simulink model "ANF"  (R2017b)
settings: Solver=VariableStepAuto  StartTime=0.0  StopTime=0.4  MaxStep=1e-4  RelTol=1e-3
libraries: powerlib x5
settings Model: Creator=Kalpit  LastModifiedBy=Kalpit

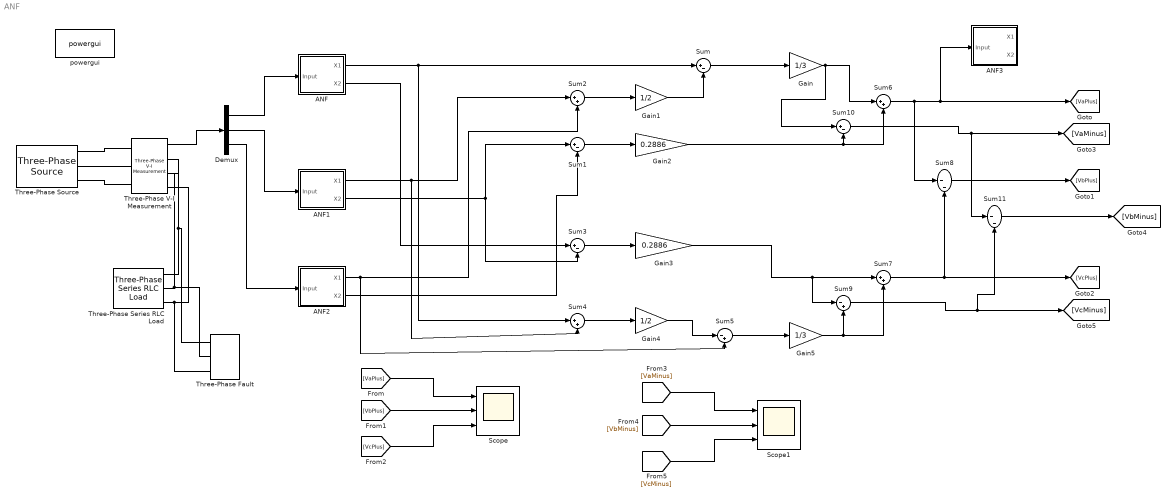
== system ANF ==
  ANF : Subsystem
  ANF1 : Subsystem
  ANF2 : Subsystem
  ANF3 : Subsystem
  Demux : Demux  Outputs=3
  Gain : Gain  Gain=1/3
  Gain1 : Gain  Gain=1/2
  Gain2 : Gain  Gain=0.2886
  Gain3 : Gain  Gain=0.2886
  Gain4 : Gain  Gain=1/2
  Gain5 : Gain  Gain=1/3
  Scope : Scope  NumInputPorts=3
  Scope1 : Scope  NumInputPorts=3
  Sum{,1,3,10} (4 alike) : Sum  Inputs=|+-
  Sum11 : Sum  Inputs=|--
  Sum{2,4,6..7} (4 alike) : Sum  Inputs=|++
  Sum5 : Sum  Inputs=|-+
  Sum8 : Sum  Inputs=|--
  Sum9 : Sum  Inputs=|-+
  Three-Phase Series RLC Load : powerlib/Elements/Three-Phase Series RLC Load  LConnTagsString=A|B|C  Configuration=Y (grounded)  NominalVoltage=415  Vabc=[1e3 1e3 1e3]  Vabcp=[1e3 1e3 1e3]  NominalFrequency=50  UnbalancedPower=off  ActivePower=10e3  InductivePower=100  CapacitivePower=100  Pabc=[10e3 9e3 11e3]  QLabc=[100 90 110]  QCabc=[100 90 110]  Pabcp=[10e3 9e3 11e3]  QLabcp=[100 90 110]  QCabcp=[100 90 110]  Measurements=None  LoadType=constant Z
  Three-Phase V-I Measurement : powerlib/Measurements/Three-Phase V-I Measurement  VoltageMeasurement=phase-to-ground  SetLabelV=off  LabelV=Vabc  Vpu=off  VpuLL=off  CurrentMeasurement=no  SetLabelI=off  LabelI=Iabc  Ipu=off  Pbase=100e6  Vbase=1  OutputType=Complex  PhasorSimulation=off  PSBequivalent=0
  Three-Phase Fault : powerlib/Elements/Three-Phase Fault  InitialStates=0  FaultA=on  FaultB=off  FaultC=on  GroundFault=on  SwitchTimes=0.2  External=off  SwitchStatus=NaN  FaultResistance=0.001  GroundResistance=0.01  SnubberResistance=1e6  SnubberCapacitance=inf  Measurements=None
  Three-Phase Source : powerlib/Electrical Sources/Three-Phase Source  InternalConnection=Yg  VoltagePhases=off  Voltage=415  PhaseAngle=0  Voltage_phases=[25e3 25e3 25e3]/sqrt(3)  PhaseAngles_phases=[0 -120 +120]  Frequency=50  NonIdealSource=on  SpecifyImpedance=off  Resistance=0.8929  Inductance=16.58e-3  ShortCircuitLevel=100e6  BaseVoltage=25e3  XRratio=7  BusType=swing  Pref=10e3  Qref=0  Prefabc=[10e3, 10e3, 10e3]  Qrefabc=[0, 0, 0]  Qmin=-inf  Qmax=inf
  powergui : powerlib/powergui  Priority=1  SimulationMode=Continuous  SampleTime=50e-6  frequency=60  Iterations=50  frequencyindice=50  Pbase=100e6  ErrMax=1e-4  UnitsV=kV  UnitsW=MW  buscounter=0  FunctionMessages=off  echomessages=off  EnableUseOfTLC=off  CurrentSourceSwitches=off  DisableSnubberDevices=off  DisableRonSwitches=off  DisableVfSwitches=off  DisplayEquations=off  SolverType=Tustin/Backward Euler (TBE)  Interpol=off  ExternalGateDelay=off  methode=off  Ts=100  x0status=blocks  SPID=on  SwTol=0  HookPort=off  RestoreLinks=warning  ResistiveCurrentMeasurement=off  Frange=[0:2:500]  Ylog=off  Xlog=on  ShowGrid=off  save=off  variable=ZData  structure=0  ZoomFFT=off  StartTime=0.0  cycles=1  DisplayStyle=1  fundamental=60  FreqAxis=off  MaxFrequency=1000  frequencyindicesteady=1  RmsSteady=1  display=off
  wires:
  Sum/1 -> Gain/1
  Gain1/1 -> Sum/2
  Sum2/1 -> Gain1/1
  ANF1/1(X1) -> Sum4/2, Sum2/1
  ANF/2(X2) -> Sum3/1
  ANF1/2(X2) -> Sum1/1, Sum3/2
  ANF2/1(X1) -> Sum5/2, Sum2/2
  ANF2/2(X2) -> Sum1/2
  Sum1/1 -> Gain2/1
  Sum3/1 -> Gain3/1
  Gain4/1 -> Sum5/1
  Sum5/1 -> Gain5/1
  Sum7/1 -> [VcPlus], Sum8/2
  Gain3/1 -> Sum9/1, Sum7/1
  Gain2/1 -> Sum10/2, Sum6/2
  Gain/1 -> Sum10/1, Sum6/1
  Gain5/1 -> Sum9/2, Sum7/2
  Sum8/1 -> [VbPlus]
  Sum10/1 -> Sum11/1, [VaMinus]
  Sum9/1 -> Sum11/2, [VcMinus]
  Sum11/1 -> [VbMinus]
  Sum4/1 -> Gain4/1
  Demux/1 -> ANF/1(Input)
  Demux/2 -> ANF1/1(Input)
  Demux/3 -> ANF2/1(Input)
  Three-Phase V-I Measurement/1 -> Demux/1
  [VaPlus] -> Scope/1
  [VbPlus] -> Scope/2
  [VcPlus] -> Scope/3
  ANF/1(X1) -> Sum4/1, Sum/1
  [VcMinus] -> Scope1/3
  [VbMinus] -> Scope1/2
  [VaMinus] -> Scope1/1
  Sum6/1 -> Sum8/1, ANF3/1(Input), [VaPlus]
  connections:
  Three-Phase V-I Measurement/LConn2 -- Three-Phase Source/RConn2
  Three-Phase Source/RConn1 -- Three-Phase V-I Measurement/LConn1
  Three-Phase Source/RConn3 -- Three-Phase V-I Measurement/LConn3
  Three-Phase Series RLC Load/LConn1 -- Three-Phase Fault/LConn1 -- Three-Phase V-I Measurement/RConn1
  Three-Phase V-I Measurement/RConn2 -- Three-Phase Fault/LConn2 -- Three-Phase Series RLC Load/LConn2
  Three-Phase V-I Measurement/RConn3 -- Three-Phase Fault/LConn3 -- Three-Phase Series RLC Load/LConn3

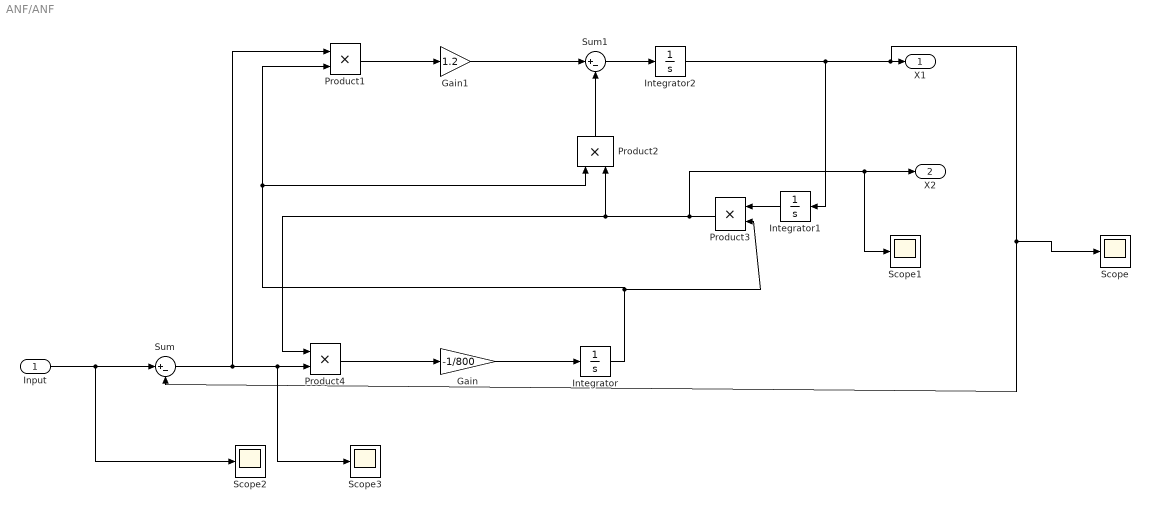
== system ANF/ANF ==
  Input : Inport
  Gain : Gain  Gain=-1/800
  Gain1 : Gain  Gain=1.2
  Integrator : Integrator  InitialCondition=100*pi
  Integrator1 : Integrator
  Integrator2 : Integrator
  Product{1..4} (4 alike) : Product
  Scope{,1..3} (4 alike) : Scope
  Sum : Sum  Inputs=|+-
  Sum1 : Sum  Inputs=|+-
  X1 : Outport
  X2 : Outport  Port=2
  wires:
  Sum1/1 -> Integrator2/1
  Sum/1 -> Product1/1, Scope3/1, Product4/2
  Product4/1 -> Gain/1
  Input/1 -> Scope2/1, Sum/1
  Integrator1/1 -> Product3/1
  Integrator2/1 -> Scope/1, Sum/2, X1/1, Integrator1/1
  Integrator/1 -> Product3/2, Product2/1, Product1/2
  Product3/1 -> Scope1/1, X2/1, Product4/1, Product2/2
  Product1/1 -> Gain1/1
  Product2/1 -> Sum1/2
  Gain/1 -> Integrator/1
  Gain1/1 -> Sum1/1

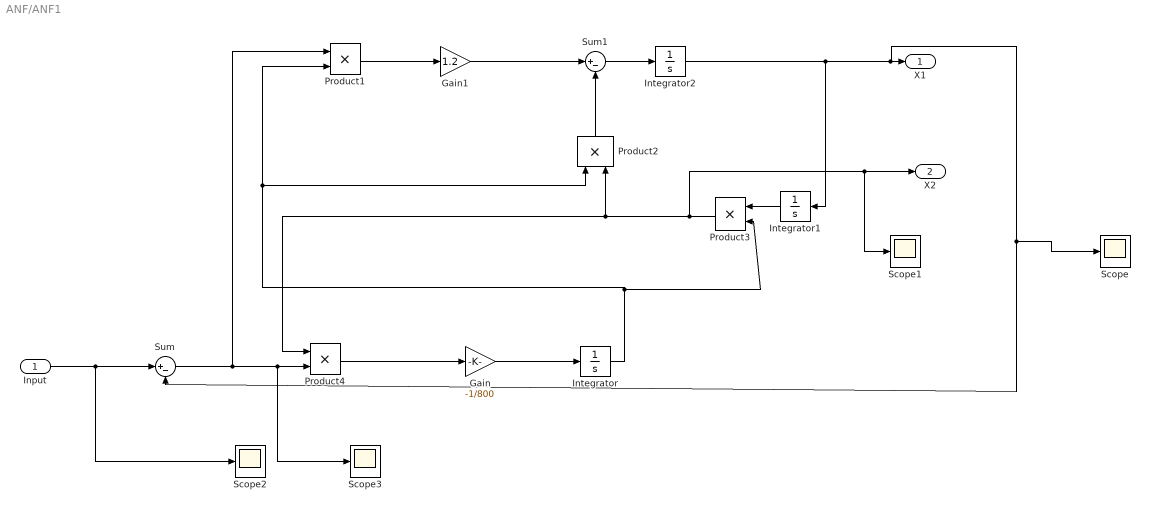
== system ANF/ANF1 ==
  Input : Inport
  Gain : Gain  Gain=-1/800
  Gain1 : Gain  Gain=1.2
  Integrator : Integrator  InitialCondition=100*pi - (2*pi/3)
  Integrator1 : Integrator
  Integrator2 : Integrator
  Product{1..4} (4 alike) : Product
  Scope{,1..3} (4 alike) : Scope
  Sum : Sum  Inputs=|+-
  Sum1 : Sum  Inputs=|+-
  X1 : Outport
  X2 : Outport  Port=2
  wires:
  Gain1/1 -> Sum1/1
  Gain/1 -> Integrator/1
  Product2/1 -> Sum1/2
  Product1/1 -> Gain1/1
  Product3/1 -> Product2/2, Product4/1, X2/1, Scope1/1
  Integrator/1 -> Product1/2, Product2/1, Product3/2
  Integrator2/1 -> Integrator1/1, X1/1, Sum/2, Scope/1
  Integrator1/1 -> Product3/1
  Input/1 -> Sum/1, Scope2/1
  Product4/1 -> Gain/1
  Sum/1 -> Product4/2, Scope3/1, Product1/1
  Sum1/1 -> Integrator2/1

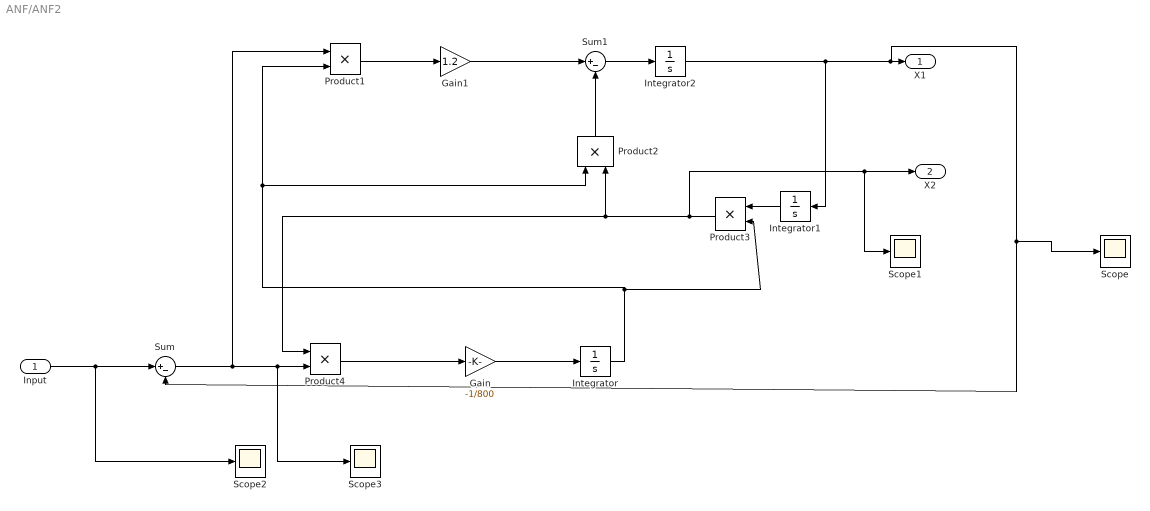
== system ANF/ANF2 ==
  Input : Inport
  Gain : Gain  Gain=-1/800
  Gain1 : Gain  Gain=1.2
  Integrator : Integrator  InitialCondition=100*pi + (2*pi/3)
  Integrator1 : Integrator
  Integrator2 : Integrator
  Product{1..4} (4 alike) : Product
  Scope{,1..3} (4 alike) : Scope
  Sum : Sum  Inputs=|+-
  Sum1 : Sum  Inputs=|+-
  X1 : Outport
  X2 : Outport  Port=2
  wires:
  Sum1/1 -> Integrator2/1
  Sum/1 -> Product1/1, Scope3/1, Product4/2
  Product4/1 -> Gain/1
  Input/1 -> Scope2/1, Sum/1
  Integrator1/1 -> Product3/1
  Integrator2/1 -> Scope/1, Sum/2, X1/1, Integrator1/1
  Integrator/1 -> Product3/2, Product2/1, Product1/2
  Product3/1 -> Scope1/1, X2/1, Product4/1, Product2/2
  Product1/1 -> Gain1/1
  Product2/1 -> Sum1/2
  Gain/1 -> Integrator/1
  Gain1/1 -> Sum1/1

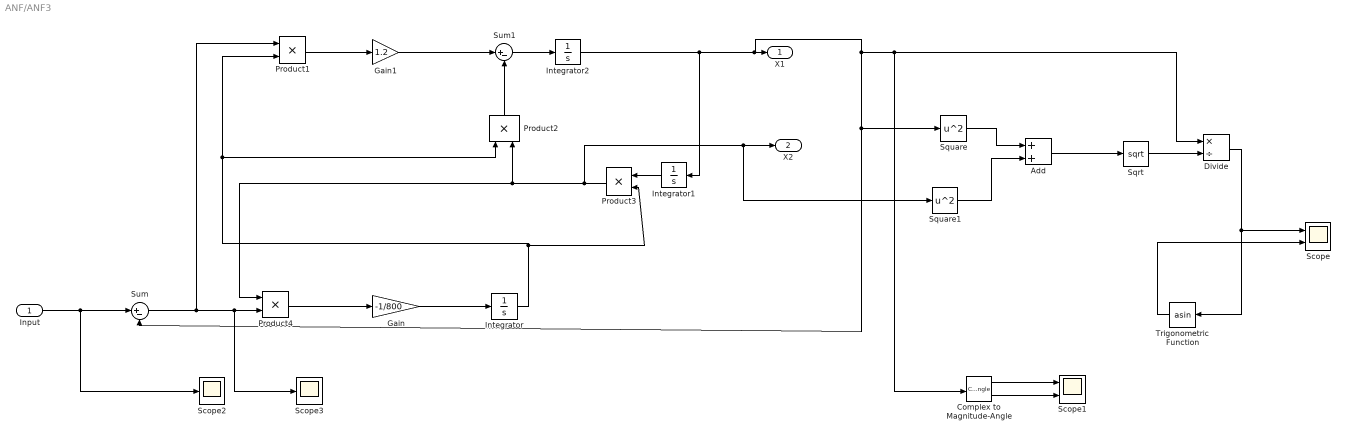
== system ANF/ANF3 ==
  Input : Inport
  Add : Sum
  Complex to Magnitude-Angle : ComplexToMagnitudeAngle
  Divide : Product  Inputs=*/
  Gain : Gain  Gain=-1/800
  Gain1 : Gain  Gain=1.2
  Integrator : Integrator  InitialCondition=100*pi
  Integrator1 : Integrator
  Integrator2 : Integrator
  Product{1..4} (4 alike) : Product
  Scope : Scope  NumInputPorts=2
  Scope1 : Scope  NumInputPorts=2
  Scope2 : Scope
  Scope3 : Scope
  Sqrt : Sqrt  SaturateOnIntegerOverflow=on
  Square : Math  Operator=square  RndMeth=Zero  SaturateOnIntegerOverflow=on
  Square1 : Math  Operator=square  RndMeth=Zero  SaturateOnIntegerOverflow=on
  Sum : Sum  Inputs=|+-
  Sum1 : Sum  Inputs=|+-
  Trigonometric Function : Trigonometry  Operator=asin
  X1 : Outport
  X2 : Outport  Port=2
  wires:
  Gain1/1 -> Sum1/1
  Gain/1 -> Integrator/1
  Product2/1 -> Sum1/2
  Product1/1 -> Gain1/1
  Product3/1 -> Product2/2, Product4/1, Square1/1, X2/1
  Integrator/1 -> Product1/2, Product2/1, Product3/2
  Integrator1/1 -> Product3/1
  Input/1 -> Sum/1, Scope2/1
  Product4/1 -> Gain/1
  Sum/1 -> Product4/2, Scope3/1, Product1/1
  Sum1/1 -> Integrator2/1
  Square/1 -> Add/1
  Square1/1 -> Add/2
  Add/1 -> Sqrt/1
  Integrator2/1 -> Integrator1/1, X1/1, Complex to Magnitude-Angle/1, Divide/1, Sum/2, Square/1
  Sqrt/1 -> Divide/2
  Divide/1 -> Trigonometric Function/1, Scope/1
  Trigonometric Function/1 -> Scope/2
  Complex to Magnitude-Angle/2 -> Scope1/2
  Complex to Magnitude-Angle/1 -> Scope1/1
